simulink model "case3"  (R2024b)
settings: Solver=FixedStepAuto  StartTime=0  StopTime=1  FixedStep=1e-7  RelTol=1e-3
values from neighbouring files (symbols this model uses):
  SG_D_1_D = 0.01056    [IEEE9_case_parameters.m]    (also in case1_parameters.m; case2_parameters.m; case3_parameters.m; case4_parameters.m)
  SG_D_1_EnableSaturation = 0    [IEEE9_case_parameters.m]    (also in case1_parameters.m; case2_parameters.m; case3_parameters.m; case4_parameters.m)
  SG_D_1_f0 = 60    [IEEE9_case_parameters.m]    (also in case1_parameters.m; case2_parameters.m; case3_parameters.m; case4_parameters.m)
  SG_D_1_H = 7.5    [IEEE9_case_parameters.m]    (also in case1_parameters.m; case2_parameters.m; case3_parameters.m; case4_parameters.m)
  SG_D_1_K_A = 20    [IEEE9_case_parameters.m]    (also in case1_parameters.m; case2_parameters.m; case3_parameters.m; case4_parameters.m)
  SG_D_1_K_E = 1.000000e+1    (= 10)    [IEEE9_case_parameters.m]    (also in case1_parameters.m; case2_parameters.m; case3_parameters.m; case4_parameters.m)
  SG_D_1_K_F = 2.363    [IEEE9_case_parameters.m]    (also in case1_parameters.m; case2_parameters.m; case3_parameters.m; case4_parameters.m)
  SG_D_1_K_s = 0.5    [IEEE9_case_parameters.m]    (also in case1_parameters.m = 5; case2_parameters.m = 5; case3_parameters.m = 5; case4_parameters.m = 5)
  SG_D_1_R_a = 0.001088    [IEEE9_case_parameters.m]    (also in case1_parameters.m; case2_parameters.m; case3_parameters.m; case4_parameters.m)
  SG_D_1_S_A = 1    [IEEE9_case_parameters.m]    (also in case1_parameters.m; case2_parameters.m; case3_parameters.m; case4_parameters.m)
  SG_D_1_S_B = 0.103    [IEEE9_case_parameters.m]    (also in case1_parameters.m; case2_parameters.m; case3_parameters.m; case4_parameters.m)
  SG_D_1_S_N = 10.659857    [IEEE9_case_parameters.m]    (also in case1_parameters.m; case2_parameters.m; case3_parameters.m; case4_parameters.m)
  SG_D_1_SpeedPara = 200    [IEEE9_case_parameters.m]    (also in case1_parameters.m; case2_parameters.m; case3_parameters.m; case4_parameters.m)
  SG_D_1_T_0 = 0.720173    [IEEE9_case_parameters.m]    (also in case1_parameters.m = 0.755522; case2_parameters.m = 0.808931; case3_parameters.m = 0.869402; case4_parameters.m = 0.729316)
  SG_D_1_T_1 = 0.3    [IEEE9_case_parameters.m]    (also in case1_parameters.m; case2_parameters.m; case3_parameters.m; case4_parameters.m)
  SG_D_1_T_2 = 0.05    [IEEE9_case_parameters.m]    (also in case1_parameters.m; case2_parameters.m; case3_parameters.m; case4_parameters.m)
  SG_D_1_T_3 = 0.02    [IEEE9_case_parameters.m]    (also in case1_parameters.m; case2_parameters.m; case3_parameters.m; case4_parameters.m)
  SG_D_1_T_4 = 0.005    [IEEE9_case_parameters.m]    (also in case1_parameters.m; case2_parameters.m; case3_parameters.m; case4_parameters.m)
  SG_D_1_T_A = 0.02    [IEEE9_case_parameters.m]    (also in case1_parameters.m; case2_parameters.m; case3_parameters.m; case4_parameters.m)
  SG_D_1_T_dd = 8.000000e+0    (= 8)    [IEEE9_case_parameters.m]    (also in case1_parameters.m; case2_parameters.m; case3_parameters.m; case4_parameters.m)
  SG_D_1_T_ddd = 0.04    [IEEE9_case_parameters.m]    (also in case1_parameters.m; case2_parameters.m; case3_parameters.m; case4_parameters.m)
  SG_D_1_T_E = 0.314    [IEEE9_case_parameters.m]    (also in case1_parameters.m; case2_parameters.m; case3_parameters.m; case4_parameters.m)
  SG_D_1_T_F = 0.35    [IEEE9_case_parameters.m]    (also in case1_parameters.m; case2_parameters.m; case3_parameters.m; case4_parameters.m)
  SG_D_1_T_qd = 0.8    [IEEE9_case_parameters.m]    (also in case1_parameters.m; case2_parameters.m; case3_parameters.m; case4_parameters.m)
  SG_D_1_T_qdd = 0.02    [IEEE9_case_parameters.m]    (also in case1_parameters.m; case2_parameters.m; case3_parameters.m; case4_parameters.m)
  SG_D_1_T_speed = 0.1    [IEEE9_case_parameters.m]    (also in case1_parameters.m = 200; case2_parameters.m = 200; case3_parameters.m = 200; case4_parameters.m = 200)
  SG_D_1_T_w = 0.5    [IEEE9_case_parameters.m]    (also in case1_parameters.m; case2_parameters.m; case3_parameters.m; case4_parameters.m)
  SG_D_1_V_ref = 1.990276    [IEEE9_case_parameters.m]    (also in case1_parameters.m = 2.042296; case2_parameters.m = 2.051388; case3_parameters.m = 2.089584; case4_parameters.m = 2.01845)
  SG_D_1_w_ref = 376.991118    [IEEE9_case_parameters.m]    (also in case1_parameters.m; case2_parameters.m; case3_parameters.m; case4_parameters.m)
  SG_D_1_wb = 6.000000e+1    (= 60)    [IEEE9_case_parameters.m]    (also in case1_parameters.m; case2_parameters.m; case3_parameters.m; case4_parameters.m)
  SG_D_1_x_d = 1.9    [IEEE9_case_parameters.m]    (also in case1_parameters.m; case2_parameters.m; case3_parameters.m; case4_parameters.m)
  SG_D_1_x_dd = 0.302    [IEEE9_case_parameters.m]    (also in case1_parameters.m; case2_parameters.m; case3_parameters.m; case4_parameters.m)
  SG_D_1_x_ddd = 0.204    [IEEE9_case_parameters.m]    (also in case1_parameters.m; case2_parameters.m; case3_parameters.m; case4_parameters.m)
  SG_D_1_x_l = 0.05    [IEEE9_case_parameters.m]    (also in case1_parameters.m; case2_parameters.m; case3_parameters.m; case4_parameters.m)
  SG_D_1_x_q = 1.3    [IEEE9_case_parameters.m]    (also in case1_parameters.m; case2_parameters.m; case3_parameters.m; case4_parameters.m)
  SG_D_1_x_qd = 0.5    [IEEE9_case_parameters.m]    (also in case1_parameters.m; case2_parameters.m; case3_parameters.m; case4_parameters.m)
  SG_D_1_x_qdd = 0.3    [IEEE9_case_parameters.m]    (also in case1_parameters.m; case2_parameters.m; case3_parameters.m; case4_parameters.m)
  SG_D_2_D = 0.02    [IEEE9_case_parameters.m]    (also in case1_parameters.m; case2_parameters.m; case3_parameters.m; case4_parameters.m)
  SG_D_2_EnableSaturation = 0    [IEEE9_case_parameters.m]    (also in case1_parameters.m; case2_parameters.m; case3_parameters.m; case4_parameters.m)
  SG_D_2_f0 = 60    [IEEE9_case_parameters.m]    (also in case1_parameters.m; case2_parameters.m; case3_parameters.m; case4_parameters.m)
  SG_D_2_H = 8.000000e+0    (= 8)    [IEEE9_case_parameters.m]    (also in case1_parameters.m; case2_parameters.m; case3_parameters.m; case4_parameters.m)
  SG_D_2_K_A = 20    [IEEE9_case_parameters.m]    (also in case1_parameters.m; case2_parameters.m; case3_parameters.m; case4_parameters.m)
  SG_D_2_K_E = 1.000000e+1    (= 10)    [IEEE9_case_parameters.m]    (also in case1_parameters.m; case2_parameters.m; case3_parameters.m; case4_parameters.m)
  SG_D_2_K_F = 2.363    [IEEE9_case_parameters.m]    (also in case1_parameters.m; case2_parameters.m; case3_parameters.m; case4_parameters.m)
  SG_D_2_K_s = 0.5    [IEEE9_case_parameters.m]    (also in case1_parameters.m = 4; case2_parameters.m = 4; case3_parameters.m = 4; case4_parameters.m = 4)
  SG_D_2_R_a = 0.001088    [IEEE9_case_parameters.m]    (also in case1_parameters.m; case2_parameters.m; case3_parameters.m; case4_parameters.m)
  SG_D_2_S_A = 1    [IEEE9_case_parameters.m]    (also in case1_parameters.m; case2_parameters.m; case3_parameters.m; case4_parameters.m)
  SG_D_2_S_B = 0.103    [IEEE9_case_parameters.m]    (also in case1_parameters.m; case2_parameters.m; case3_parameters.m; case4_parameters.m)
  SG_D_2_S_N = 10.659857    [IEEE9_case_parameters.m]    (also in case1_parameters.m; case2_parameters.m; case3_parameters.m; case4_parameters.m)
  SG_D_2_SpeedPara = 200    [IEEE9_case_parameters.m]    (also in case1_parameters.m; case2_parameters.m; case3_parameters.m; case4_parameters.m)
  SG_D_2_T_0 = 1.632913    [IEEE9_case_parameters.m]    (also in case1_parameters.m = 1.632925; case2_parameters.m = 1.632915; case3_parameters.m = 1.632914; case4_parameters.m = 1.632927)
  SG_D_2_T_1 = 0.2    [IEEE9_case_parameters.m]    (also in case1_parameters.m; case2_parameters.m; case3_parameters.m; case4_parameters.m)
  SG_D_2_T_2 = 0.05    [IEEE9_case_parameters.m]    (also in case1_parameters.m; case2_parameters.m; case3_parameters.m; case4_parameters.m)
  SG_D_2_T_3 = 0.02    [IEEE9_case_parameters.m]    (also in case1_parameters.m; case2_parameters.m; case3_parameters.m; case4_parameters.m)
  SG_D_2_T_4 = 0.005    [IEEE9_case_parameters.m]    (also in case1_parameters.m; case2_parameters.m; case3_parameters.m; case4_parameters.m)
  SG_D_2_T_A = 0.02    [IEEE9_case_parameters.m]    (also in case1_parameters.m; case2_parameters.m; case3_parameters.m; case4_parameters.m)
  SG_D_2_T_dd = 7.9    [IEEE9_case_parameters.m]    (also in case1_parameters.m; case2_parameters.m; case3_parameters.m; case4_parameters.m)
  SG_D_2_T_ddd = 0.04    [IEEE9_case_parameters.m]    (also in case1_parameters.m; case2_parameters.m; case3_parameters.m; case4_parameters.m)
  SG_D_2_T_E = 0.314    [IEEE9_case_parameters.m]    (also in case1_parameters.m; case2_parameters.m; case3_parameters.m; case4_parameters.m)
  SG_D_2_T_F = 0.35    [IEEE9_case_parameters.m]    (also in case1_parameters.m; case2_parameters.m; case3_parameters.m; case4_parameters.m)
  SG_D_2_T_qd = 0.8    [IEEE9_case_parameters.m]    (also in case1_parameters.m; case2_parameters.m; case3_parameters.m; case4_parameters.m)
  SG_D_2_T_qdd = 0.015    [IEEE9_case_parameters.m]    (also in case1_parameters.m; case2_parameters.m; case3_parameters.m; case4_parameters.m)
  SG_D_2_T_speed = 0.1    [IEEE9_case_parameters.m]    (also in case1_parameters.m = 150; case2_parameters.m = 150; case3_parameters.m = 150; case4_parameters.m = 150)
  SG_D_2_T_w = 0.35    [IEEE9_case_parameters.m]    (also in case1_parameters.m; case2_parameters.m; case3_parameters.m; case4_parameters.m)
  SG_D_2_V_ref = 2.58547    [IEEE9_case_parameters.m]    (also in case1_parameters.m = 2.597896; case2_parameters.m = 2.587136; case3_parameters.m = 2.586042; case4_parameters.m = 2.599679)
  SG_D_2_w_ref = 376.991118    [IEEE9_case_parameters.m]    (also in case1_parameters.m; case2_parameters.m; case3_parameters.m; case4_parameters.m)
  SG_D_2_wb = 6.000000e+1    (= 60)    [IEEE9_case_parameters.m]    (also in case1_parameters.m; case2_parameters.m; case3_parameters.m; case4_parameters.m)
  SG_D_2_x_d = 1.8    [IEEE9_case_parameters.m]    (also in case1_parameters.m; case2_parameters.m; case3_parameters.m; case4_parameters.m)
  SG_D_2_x_dd = 0.302    [IEEE9_case_parameters.m]    (also in case1_parameters.m; case2_parameters.m; case3_parameters.m; case4_parameters.m)
  SG_D_2_x_ddd = 0.204    [IEEE9_case_parameters.m]    (also in case1_parameters.m; case2_parameters.m; case3_parameters.m; case4_parameters.m)
  SG_D_2_x_l = 0.05    [IEEE9_case_parameters.m]    (also in case1_parameters.m; case2_parameters.m; case3_parameters.m; case4_parameters.m)
  SG_D_2_x_q = 1.25    [IEEE9_case_parameters.m]    (also in case1_parameters.m; case2_parameters.m; case3_parameters.m; case4_parameters.m)
  SG_D_2_x_qd = 0.5    [IEEE9_case_parameters.m]    (also in case1_parameters.m; case2_parameters.m; case3_parameters.m; case4_parameters.m)
  SG_D_2_x_qdd = 0.3    [IEEE9_case_parameters.m]    (also in case1_parameters.m; case2_parameters.m; case3_parameters.m; case4_parameters.m)
  SG_D_3_D = 0.02    [IEEE9_case_parameters.m]    (also in case1_parameters.m; case2_parameters.m; case3_parameters.m; case4_parameters.m)
  SG_D_3_EnableSaturation = 0    [IEEE9_case_parameters.m]    (also in case1_parameters.m; case2_parameters.m; case3_parameters.m; case4_parameters.m)
  SG_D_3_f0 = 60    [IEEE9_case_parameters.m]    (also in case1_parameters.m; case2_parameters.m; case3_parameters.m; case4_parameters.m)
  SG_D_3_H = 7.7    [IEEE9_case_parameters.m]    (also in case1_parameters.m; case2_parameters.m; case3_parameters.m; case4_parameters.m)
  SG_D_3_K_A = 20    [IEEE9_case_parameters.m]    (also in case1_parameters.m; case2_parameters.m; case3_parameters.m; case4_parameters.m)
  SG_D_3_K_E = 1.000000e+1    (= 10)    [IEEE9_case_parameters.m]    (also in case1_parameters.m; case2_parameters.m; case3_parameters.m; case4_parameters.m)
  SG_D_3_K_F = 2.363    [IEEE9_case_parameters.m]    (also in case1_parameters.m; case2_parameters.m; case3_parameters.m; case4_parameters.m)
  SG_D_3_K_s = 0.2    [IEEE9_case_parameters.m]    (also in case1_parameters.m = 2; case2_parameters.m = 2; case3_parameters.m = 2; case4_parameters.m = 2)
  SG_D_3_R_a = 0.001088    [IEEE9_case_parameters.m]    (also in case1_parameters.m; case2_parameters.m; case3_parameters.m; case4_parameters.m)
  SG_D_3_S_A = 1    [IEEE9_case_parameters.m]    (also in case1_parameters.m; case2_parameters.m; case3_parameters.m; case4_parameters.m)
  SG_D_3_S_B = 0.103    [IEEE9_case_parameters.m]    (also in case1_parameters.m; case2_parameters.m; case3_parameters.m; case4_parameters.m)
  SG_D_3_S_N = 10.659857    [IEEE9_case_parameters.m]    (also in case1_parameters.m; case2_parameters.m; case3_parameters.m; case4_parameters.m)
  SG_D_3_SpeedPara = 200    [IEEE9_case_parameters.m]    (also in case1_parameters.m; case2_parameters.m; case3_parameters.m; case4_parameters.m)
  SG_D_3_T_0 = 0.850788    [IEEE9_case_parameters.m]    (also in case1_parameters.m = 0.850786; case2_parameters.m = 0.850787; case3_parameters.m; case4_parameters.m = 0.850786)
  SG_D_3_T_1 = 0.2    [IEEE9_case_parameters.m]    (also in case1_parameters.m; case2_parameters.m; case3_parameters.m; case4_parameters.m)
  SG_D_3_T_2 = 0.05    [IEEE9_case_parameters.m]    (also in case1_parameters.m; case2_parameters.m; case3_parameters.m; case4_parameters.m)
  SG_D_3_T_3 = 0.02    [IEEE9_case_parameters.m]    (also in case1_parameters.m; case2_parameters.m; case3_parameters.m; case4_parameters.m)
  SG_D_3_T_4 = 0.005    [IEEE9_case_parameters.m]    (also in case1_parameters.m; case2_parameters.m; case3_parameters.m; case4_parameters.m)
  SG_D_3_T_A = 0.02    [IEEE9_case_parameters.m]    (also in case1_parameters.m; case2_parameters.m; case3_parameters.m; case4_parameters.m)
  SG_D_3_T_dd = 8.1    [IEEE9_case_parameters.m]    (also in case1_parameters.m; case2_parameters.m; case3_parameters.m; case4_parameters.m)
  SG_D_3_T_ddd = 0.04    [IEEE9_case_parameters.m]    (also in case1_parameters.m; case2_parameters.m; case3_parameters.m; case4_parameters.m)
  SG_D_3_T_E = 0.314    [IEEE9_case_parameters.m]    (also in case1_parameters.m; case2_parameters.m; case3_parameters.m; case4_parameters.m)
  SG_D_3_T_F = 0.35    [IEEE9_case_parameters.m]    (also in case1_parameters.m; case2_parameters.m; case3_parameters.m; case4_parameters.m)
  SG_D_3_T_qd = 0.8    [IEEE9_case_parameters.m]    (also in case1_parameters.m; case2_parameters.m; case3_parameters.m; case4_parameters.m)
  SG_D_3_T_qdd = 0.015    [IEEE9_case_parameters.m]    (also in case1_parameters.m; case2_parameters.m; case3_parameters.m; case4_parameters.m)
  SG_D_3_T_speed = 0.1    [IEEE9_case_parameters.m]    (also in case1_parameters.m = 180; case2_parameters.m = 180; case3_parameters.m = 180; case4_parameters.m = 180)
  SG_D_3_T_w = 0.4    [IEEE9_case_parameters.m]    (also in case1_parameters.m; case2_parameters.m; case3_parameters.m; case4_parameters.m)
  SG_D_3_V_ref = 1.892727    [IEEE9_case_parameters.m]    (also in case1_parameters.m = 1.906439; case2_parameters.m = 1.895535; case3_parameters.m = 1.892105; case4_parameters.m = 1.906598)
  SG_D_3_w_ref = 376.991118    [IEEE9_case_parameters.m]    (also in case1_parameters.m; case2_parameters.m; case3_parameters.m; case4_parameters.m)
  SG_D_3_wb = 6.000000e+1    (= 60)    [IEEE9_case_parameters.m]    (also in case1_parameters.m; case2_parameters.m; case3_parameters.m; case4_parameters.m)
  SG_D_3_x_d = 1.85    [IEEE9_case_parameters.m]    (also in case1_parameters.m; case2_parameters.m; case3_parameters.m; case4_parameters.m)
  SG_D_3_x_dd = 0.302    [IEEE9_case_parameters.m]    (also in case1_parameters.m; case2_parameters.m; case3_parameters.m; case4_parameters.m)
  SG_D_3_x_ddd = 0.204    [IEEE9_case_parameters.m]    (also in case1_parameters.m; case2_parameters.m; case3_parameters.m; case4_parameters.m)
  SG_D_3_x_l = 0.05    [IEEE9_case_parameters.m]    (also in case1_parameters.m; case2_parameters.m; case3_parameters.m; case4_parameters.m)
  SG_D_3_x_q = 1.2    [IEEE9_case_parameters.m]    (also in case1_parameters.m; case2_parameters.m; case3_parameters.m; case4_parameters.m)
  SG_D_3_x_qd = 0.5    [IEEE9_case_parameters.m]    (also in case1_parameters.m; case2_parameters.m; case3_parameters.m; case4_parameters.m)
  SG_D_3_x_qdd = 0.3    [IEEE9_case_parameters.m]    (also in case1_parameters.m; case2_parameters.m; case3_parameters.m; case4_parameters.m)
(part 1 of 12)
settings Model: Creator=Greg  LastModifiedBy=Greg

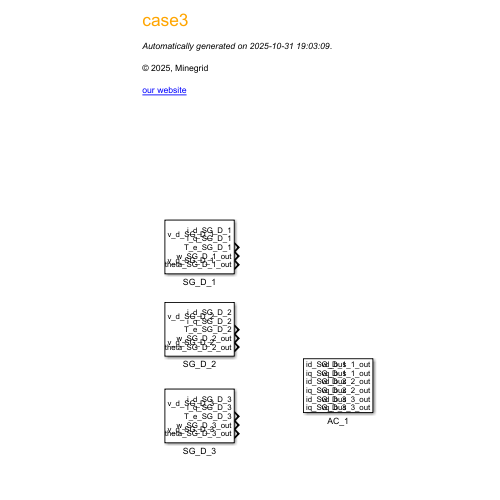
[thumbnail: Simulink's stored preview of the top-level diagram]
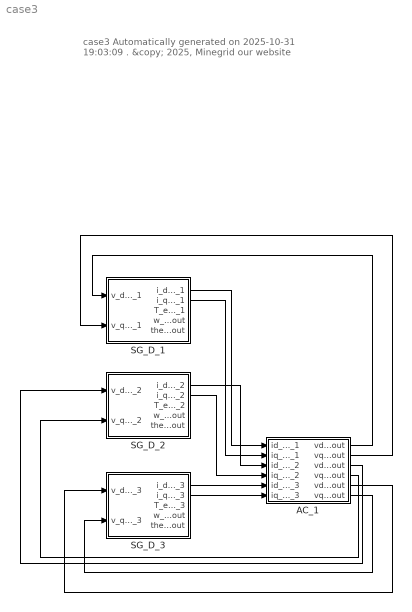
== system case3 ==
  note: case3
      | Automatically generated on 2025-10-31 19:03:09 .
      | &copy; 2025, Minegrid
      | our website
  AC_1 : Subsystem  mask(AC_1){}
      mask help: Parameters Interface of AC_1
  SG_D_1 : Subsystem  mask(SG_D_1){T_0=SG_D_1_T_0, w_ref=SG_D_1_w_ref, V_ref=SG_D_1_V_ref, x_d=SG_D_1_x_d, x_dd=SG_D_1_x_dd, x_ddd=SG_D_1_x_ddd, x_q=SG_D_1_x_q, x_qd=SG_D_1_x_qd, x_qdd=SG_D_1_x_qdd, x_l=SG_D_1_x_l, R_a=SG_D_1_R_a, T_dd=SG_D_1_T_dd, T_ddd=SG_D_1_T_ddd, T_qd=SG_D_1_T_qd, T_qdd=SG_D_1_T_qdd, H=SG_D_1_H, D=SG_D_1_D, SpeedPara=SG_D_1_SpeedPara, K_A=SG_D_1_K_A, EnableSaturation=SG_D_1_EnableSaturation, f0=SG_D_1_f0, T_speed=SG_D_1_T_speed, T_E=SG_D_1_T_E, T_A=SG_D_1_T_A, T_F=SG_D_1_T_F, K_E=SG_D_1_K_E, K_F=SG_D_1_K_F, K_s=SG_D_1_K_s, T_1=SG_D_1_T_1, T_2=SG_D_1_T_2, T_3=SG_D_1_T_3, T_4=SG_D_1_T_4, T_w=SG_D_1_T_w, wb=SG_D_1_wb, S_A=SG_D_1_S_A, S_B=SG_D_1_S_B, S_N=SG_D_1_S_N}
      mask help: Parameters Interface of SG_D_1
  SG_D_2 : Subsystem  mask(SG_D_2){T_0=SG_D_2_T_0, w_ref=SG_D_2_w_ref, V_ref=SG_D_2_V_ref, x_d=SG_D_2_x_d, x_dd=SG_D_2_x_dd, x_ddd=SG_D_2_x_ddd, x_q=SG_D_2_x_q, x_qd=SG_D_2_x_qd, x_qdd=SG_D_2_x_qdd, x_l=SG_D_2_x_l, R_a=SG_D_2_R_a, T_dd=SG_D_2_T_dd, T_ddd=SG_D_2_T_ddd, T_qd=SG_D_2_T_qd, T_qdd=SG_D_2_T_qdd, H=SG_D_2_H, D=SG_D_2_D, SpeedPara=SG_D_2_SpeedPara, K_A=SG_D_2_K_A, EnableSaturation=SG_D_2_EnableSaturation, f0=SG_D_2_f0, T_speed=SG_D_2_T_speed, T_E=SG_D_2_T_E, T_A=SG_D_2_T_A, T_F=SG_D_2_T_F, K_E=SG_D_2_K_E, K_F=SG_D_2_K_F, K_s=SG_D_2_K_s, T_1=SG_D_2_T_1, T_2=SG_D_2_T_2, T_3=SG_D_2_T_3, T_4=SG_D_2_T_4, T_w=SG_D_2_T_w, wb=SG_D_2_wb, S_A=SG_D_2_S_A, S_B=SG_D_2_S_B, S_N=SG_D_2_S_N}
      mask help: Parameters Interface of SG_D_2
  SG_D_3 : Subsystem  mask(SG_D_3){T_0=SG_D_3_T_0, w_ref=SG_D_3_w_ref, V_ref=SG_D_3_V_ref, x_d=SG_D_3_x_d, x_dd=SG_D_3_x_dd, x_ddd=SG_D_3_x_ddd, x_q=SG_D_3_x_q, x_qd=SG_D_3_x_qd, x_qdd=SG_D_3_x_qdd, x_l=SG_D_3_x_l, R_a=SG_D_3_R_a, T_dd=SG_D_3_T_dd, T_ddd=SG_D_3_T_ddd, T_qd=SG_D_3_T_qd, T_qdd=SG_D_3_T_qdd, H=SG_D_3_H, D=SG_D_3_D, SpeedPara=SG_D_3_SpeedPara, K_A=SG_D_3_K_A, EnableSaturation=SG_D_3_EnableSaturation, f0=SG_D_3_f0, T_speed=SG_D_3_T_speed, T_E=SG_D_3_T_E, T_A=SG_D_3_T_A, T_F=SG_D_3_T_F, K_E=SG_D_3_K_E, K_F=SG_D_3_K_F, K_s=SG_D_3_K_s, T_1=SG_D_3_T_1, T_2=SG_D_3_T_2, T_3=SG_D_3_T_3, T_4=SG_D_3_T_4, T_w=SG_D_3_T_w, wb=SG_D_3_wb, S_A=SG_D_3_S_A, S_B=SG_D_3_S_B, S_N=SG_D_3_S_N}
      mask help: Parameters Interface of SG_D_3
  wires:
  SG_D_2/2(i_q_SG_D_2) -> AC_1/4(iq_SG_D_2)
  SG_D_1/2(i_q_SG_D_1) -> AC_1/2(iq_SG_D_1)
  SG_D_1/1(i_d_SG_D_1) -> AC_1/1(id_SG_D_1)
  SG_D_2/1(i_d_SG_D_2) -> AC_1/3(id_SG_D_2)
  AC_1/1(vd_bus_1_out) -> SG_D_1/1(v_d_SG_D_1)
  SG_D_3/1(i_d_SG_D_3) -> AC_1/5(id_SG_D_3)
  AC_1/2(vq_bus_1_out) -> SG_D_1/2(v_q_SG_D_1)
  SG_D_3/2(i_q_SG_D_3) -> AC_1/6(iq_SG_D_3)
  AC_1/3(vd_bus_2_out) -> SG_D_2/1(v_d_SG_D_2)
  AC_1/4(vq_bus_2_out) -> SG_D_2/2(v_q_SG_D_2)
  AC_1/5(vd_bus_3_out) -> SG_D_3/1(v_d_SG_D_3)
  AC_1/6(vq_bus_3_out) -> SG_D_3/2(v_q_SG_D_3)

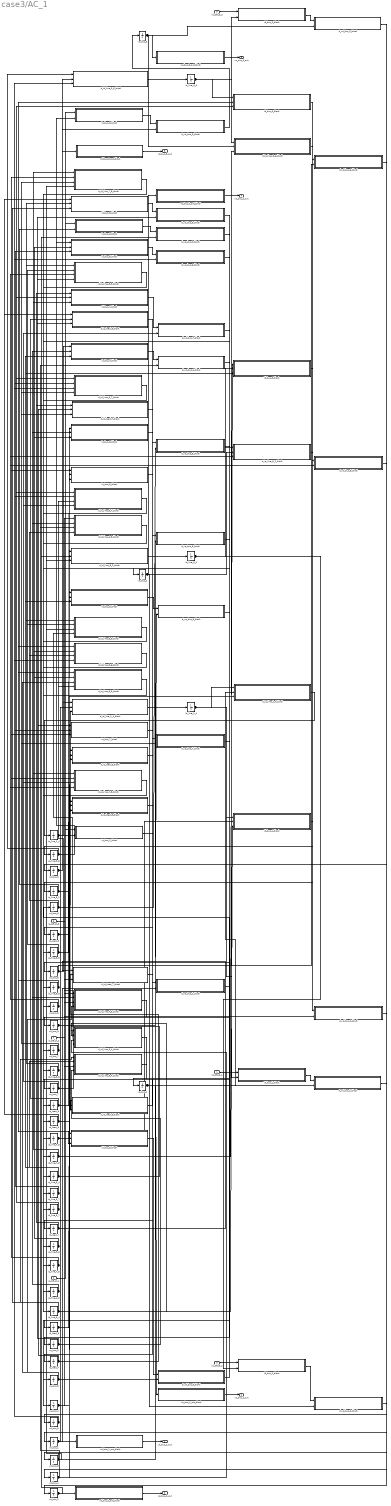
== system case3/AC_1 ==
  id_SG_D_1 : Inport
  iq_SG_D_1 : Inport  Port=2
  id_SG_D_2 : Inport  Port=3
  iq_SG_D_2 : Inport  Port=4
  id_SG_D_3 : Inport  Port=5
  iq_SG_D_3 : Inport  Port=6
  d_id_line_1_4_block : Subsystem
  d_id_line_3_6_block : Subsystem
  d_id_line_4_5_block : Subsystem
  d_id_line_5_6_block : Subsystem
  d_id_line_6_7_block : Subsystem
  d_id_line_7_8_block : Subsystem
  d_id_line_8_2_block : Subsystem
  d_id_line_8_9_block : Subsystem
  d_id_line_9_4_block : Subsystem
  d_id_load_5_block : Subsystem
  d_id_load_7_block : Subsystem
  d_id_load_9_block : Subsystem
  d_iq_line_1_4_block : Subsystem
  d_iq_line_3_6_block : Subsystem
  d_iq_line_4_5_block : Subsystem
  d_iq_line_5_6_block : Subsystem
  d_iq_line_6_7_block : Subsystem
  d_iq_line_7_8_block : Subsystem
  d_iq_line_8_2_block : Subsystem
  d_iq_line_8_9_block : Subsystem
  d_iq_line_9_4_block : Subsystem
  d_iq_load_5_block : Subsystem
  d_iq_load_7_block : Subsystem
  d_iq_load_9_block : Subsystem
  d_vd_bus_1_block : Subsystem
  d_vd_bus_2_block : Subsystem
  d_vd_bus_3_block : Subsystem
  d_vd_bus_4_block : Subsystem
  d_vd_bus_5_block : Subsystem
  d_vd_bus_6_block : Subsystem
  d_vd_bus_7_block : Subsystem
  d_vd_bus_8_block : Subsystem
  d_vd_bus_9_block : Subsystem
  d_vq_bus_1_block : Subsystem
  d_vq_bus_2_block : Subsystem
  d_vq_bus_3_block : Subsystem
  d_vq_bus_4_block : Subsystem
  d_vq_bus_5_block : Subsystem
  d_vq_bus_6_block : Subsystem
  d_vq_bus_7_block : Subsystem
  d_vq_bus_8_block : Subsystem
  d_vq_bus_9_block : Subsystem
  id_bus_1_block : Subsystem
  id_bus_2_block : Subsystem
  id_bus_3_block : Subsystem
  id_bus_4_block : Subsystem
  id_bus_5_block : Subsystem
  id_bus_6_block : Subsystem
  id_bus_7_block : Subsystem
  id_bus_8_block : Subsystem
  id_bus_9_block : Subsystem
  id_line_1_4 : Integrator  InitialCondition=0.8685
  id_line_3_6 : Integrator  InitialCondition=0.8456
  id_line_4_5 : Integrator  InitialCondition=0.3746
  id_line_5_6 : Integrator  InitialCondition=-0.5838
  id_line_6_7 : Integrator  InitialCondition=0.266
  id_line_7_8 : Integrator  InitialCondition=-0.7941
  id_line_8_2 : Integrator  InitialCondition=-1.633
  id_line_8_9 : Integrator  InitialCondition=0.8498
  id_line_9_4 : Integrator  InitialCondition=-0.4852
  id_load_5 : Integrator  InitialCondition=0.9359719094415446
  id_load_7 : Integrator  InitialCondition=1.058114773666789
  id_load_9 : Integrator  InitialCondition=1.3128275450508151
  iq_bus_1_block : Subsystem
  iq_bus_2_block : Subsystem
  iq_bus_3_block : Subsystem
  iq_bus_4_block : Subsystem
  iq_bus_5_block : Subsystem
  iq_bus_6_block : Subsystem
  iq_bus_7_block : Subsystem
  iq_bus_8_block : Subsystem
  iq_bus_9_block : Subsystem
  iq_line_1_4 : Integrator  InitialCondition=-0.239
  iq_line_3_6 : Integrator  InitialCondition=0.0944
  iq_line_4_5 : Integrator  InitialCondition=-0.0834
  iq_line_5_6 : Integrator  InitialCondition=0.0474
  iq_line_6_7 : Integrator  InitialCondition=-0.1426
  iq_line_7_8 : Integrator  InitialCondition=0.0351
  iq_line_8_2 : Integrator  InitialCondition=-0.1083
  iq_line_8_9 : Integrator  InitialCondition=-0.0829
  iq_line_9_4 : Integrator  InitialCondition=0.3203
  iq_load_5 : Integrator  InitialCondition=-0.3812628280514811
  iq_load_7 : Integrator  InitialCondition=-0.35410310514589904
  iq_load_9 : Integrator  InitialCondition=-0.6326059955985617
  vd_bus_1 : Integrator  InitialCondition=1.0
  vd_bus_1_out_block : Subsystem
  vd_bus_2 : Integrator  InitialCondition=0.9879091097107321
  vd_bus_2_out_block : Subsystem
  vd_bus_3 : Integrator  InitialCondition=0.9977645153986716
  vd_bus_3_out_block : Subsystem
  vd_bus_4 : Integrator  InitialCondition=0.9855935027057598
  vd_bus_5 : Integrator  InitialCondition=0.9707528693348056
  vd_bus_6 : Integrator  InitialCondition=1.003554613883012
  vd_bus_7 : Integrator  InitialCondition=0.9851223493487857
  vd_bus_8 : Integrator  InitialCondition=0.9949914819674712
  vd_bus_9 : Integrator  InitialCondition=0.9519187352878377
  vq_bus_1 : Integrator  InitialCondition=0.0
  vq_bus_1_out_block : Subsystem
  vq_bus_2 : Integrator  InitialCondition=0.1550341605922668
  vq_bus_2_out_block : Subsystem
  vq_bus_3 : Integrator  InitialCondition=0.06682792688131226
  vq_bus_3_out_block : Subsystem
  vq_bus_4 : Integrator  InitialCondition=-0.05234370307058784
  vq_bus_5 : Integrator  InitialCondition=-0.08688371657456954
  vq_bus_6 : Integrator  InitialCondition=0.014981980389526698
  vq_bus_7 : Integrator  InitialCondition=-0.011257511235524303
  vq_bus_8 : Integrator  InitialCondition=0.04824761170151553
  vq_bus_9 : Integrator  InitialCondition=-0.09206900230068515
  vd_bus_1_out : Outport
  vq_bus_1_out : Outport  Port=2
  vd_bus_2_out : Outport  Port=3
  vq_bus_2_out : Outport  Port=4
  vd_bus_3_out : Outport  Port=5
  vq_bus_3_out : Outport  Port=6
  wires:
  vq_bus_2_out_block/1(Blockout_vq_bus_2_out_740a9) -> vq_bus_2_out/1
  d_id_line_1_4_block/1(Blockout_d_id_line_1_4_f5e01) -> id_line_1_4/1
  iq_SG_D_3/1 -> iq_bus_3_block/1(Input_iq_SG_D_3_dee65)
  vq_bus_1/1 -> d_vd_bus_1_block/2(State_vq_bus_1_8af1f), d_iq_line_1_4_block/2(State_vq_bus_1_eaf9d), vq_bus_1_out_block/1(State_vq_bus_1_ac5cf)
  vd_bus_3_out_block/1(Blockout_vd_bus_3_out_036f2) -> vd_bus_3_out/1
  d_iq_line_8_2_block/1(Blockout_d_iq_line_8_2_aa3d3) -> iq_line_8_2/1
  d_vd_bus_4_block/1(Blockout_d_vd_bus_4_12eb5) -> vd_bus_4/1
  id_SG_D_3/1 -> id_bus_3_block/1(Input_id_SG_D_3_6c44f)
  id_SG_D_2/1 -> id_bus_2_block/1(Input_id_SG_D_2_bafef)
  vq_bus_3_out_block/1(Blockout_vq_bus_3_out_fa0c1) -> vq_bus_3_out/1
  iq_bus_8_block/1(Blockout_iq_bus_8_33408) -> d_vq_bus_8_block/1(Alge_iq_bus_8_0043b)
  iq_SG_D_2/1 -> iq_bus_2_block/1(Input_iq_SG_D_2_ed99c)
  id_SG_D_1/1 -> id_bus_1_block/1(Input_id_SG_D_1_696b1)
  id_bus_9_block/1(Blockout_id_bus_9_70dbc) -> d_vd_bus_9_block/1(Alge_id_bus_9_730d0)
  iq_SG_D_1/1 -> iq_bus_1_block/1(Input_iq_SG_D_1_691df)
  d_id_load_7_block/1(Blockout_d_id_load_7_3ef5e) -> id_load_7/1
  iq_bus_6_block/1(Blockout_iq_bus_6_95ebc) -> d_vq_bus_6_block/1(Alge_iq_bus_6_a58d3)
  id_bus_3_block/1(Blockout_id_bus_3_5b536) -> d_vd_bus_3_block/1(Alge_id_bus_3_439ad)
  id_bus_8_block/1(Blockout_id_bus_8_01350) -> d_vd_bus_8_block/1(Alge_id_bus_8_ebbc1)
  iq_bus_9_block/1(Blockout_iq_bus_9_4e4a2) -> d_vq_bus_9_block/1(Alge_iq_bus_9_e4ae9)
  id_load_9/1 -> d_id_load_9_block/1(State_id_load_9_00ea3), id_bus_9_block/1(State_id_load_9_08adc), d_iq_load_9_block/1(State_id_load_9_95b0f)
  id_bus_4_block/1(Blockout_id_bus_4_47d2f) -> d_vd_bus_4_block/1(Alge_id_bus_4_7068c)
  vd_bus_1_out_block/1(Blockout_vd_bus_1_out_2faa7) -> vd_bus_1_out/1
  vq_bus_1_out_block/1(Blockout_vq_bus_1_out_b4fc0) -> vq_bus_1_out/1
  id_bus_5_block/1(Blockout_id_bus_5_0f46c) -> d_vd_bus_5_block/1(Alge_id_bus_5_5e52c)
  iq_line_7_8/1 -> iq_bus_7_block/3(State_iq_line_7_8_95be5), iq_bus_8_block/1(State_iq_line_7_8_0aaeb), d_iq_line_7_8_block/2(State_iq_line_7_8_0ca45), d_id_line_7_8_block/2(State_iq_line_7_8_8ab2b)
  iq_bus_7_block/1(Blockout_iq_bus_7_bb486) -> d_vq_bus_7_block/1(Alge_iq_bus_7_9bcfd)
  vd_bus_6/1 -> d_id_line_5_6_block/4(State_vd_bus_6_02860), d_id_line_3_6_block/3(State_vd_bus_6_86153), d_id_line_6_7_block/3(State_vd_bus_6_9819c), d_vq_bus_6_block/2(State_vd_bus_6_2678b)
  iq_bus_2_block/1(Blockout_iq_bus_2_c2560) -> d_vq_bus_2_block/1(Alge_iq_bus_2_2abe7)
  d_vd_bus_3_block/1(Blockout_d_vd_bus_3_94704) -> vd_bus_3/1
  id_bus_7_block/1(Blockout_id_bus_7_20b6b) -> d_vd_bus_7_block/1(Alge_id_bus_7_2d419)
  id_bus_6_block/1(Blockout_id_bus_6_05d15) -> d_vd_bus_6_block/1(Alge_id_bus_6_24922)
  id_line_4_5/1 -> id_bus_4_block/2(State_id_line_4_5_71002), d_iq_line_4_5_block/1(State_id_line_4_5_24b18), d_id_line_4_5_block/1(State_id_line_4_5_125e0), id_bus_5_block/2(State_id_line_4_5_78e66)
  vd_bus_2_out_block/1(Blockout_vd_bus_2_out_79f6a) -> vd_bus_2_out/1
  id_line_9_4/1 -> d_id_line_9_4_block/1(State_id_line_9_4_02a1a), d_iq_line_9_4_block/1(State_id_line_9_4_af562), id_bus_4_block/3(State_id_line_9_4_dd8eb), id_bus_9_block/3(State_id_line_9_4_1728f)
  vq_bus_8/1 -> d_vd_bus_8_block/2(State_vq_bus_8_8405d), d_iq_line_7_8_block/4(State_vq_bus_8_3d863), d_iq_line_8_9_block/3(State_vq_bus_8_011bb), d_iq_line_8_2_block/3(State_vq_bus_8_3e61a)
  iq_bus_5_block/1(Blockout_iq_bus_5_d6d28) -> d_vq_bus_5_block/1(Alge_iq_bus_5_f83f1)
  id_line_6_7/1 -> id_bus_6_block/3(State_id_line_6_7_32134), d_id_line_6_7_block/1(State_id_line_6_7_3cec9), d_iq_line_6_7_block/1(State_id_line_6_7_cd5da), id_bus_7_block/2(State_id_line_6_7_64680)
  id_bus_2_block/1(Blockout_id_bus_2_bddd5) -> d_vd_bus_2_block/1(Alge_id_bus_2_0b6c0)
  iq_bus_4_block/1(Blockout_iq_bus_4_14ae7) -> d_vq_bus_4_block/1(Alge_iq_bus_4_f534f)
  iq_bus_3_block/1(Blockout_iq_bus_3_7f48b) -> d_vq_bus_3_block/1(Alge_iq_bus_3_adc3d)
  id_bus_1_block/1(Blockout_id_bus_1_4a65c) -> d_vd_bus_1_block/1(Alge_id_bus_1_f922c)
  iq_line_8_2/1 -> d_id_line_8_2_block/1(State_iq_line_8_2_c2450), iq_bus_2_block/2(State_iq_line_8_2_3621d), iq_bus_8_block/2(State_iq_line_8_2_60ac3)
  iq_bus_1_block/1(Blockout_iq_bus_1_cefb8) -> d_vq_bus_1_block/1(Alge_iq_bus_1_c886c)
  d_id_line_3_6_block/1(Blockout_d_id_line_3_6_3490b) -> id_line_3_6/1
  d_vq_bus_7_block/1(Blockout_d_vq_bus_7_00412) -> vq_bus_7/1
  id_line_5_6/1 -> id_bus_6_block/2(State_id_line_5_6_cc1e8), d_iq_line_5_6_block/1(State_id_line_5_6_f3a7a), id_bus_5_block/3(State_id_line_5_6_8fb3f), d_id_line_5_6_block/1(State_id_line_5_6_11d83)
  iq_line_6_7/1 -> d_iq_line_6_7_block/2(State_iq_line_6_7_f3824), iq_bus_6_block/3(State_iq_line_6_7_054b0), iq_bus_7_block/2(State_iq_line_6_7_03f81), d_id_line_6_7_block/2(State_iq_line_6_7_7db22)
  id_line_8_2/1 -> id_bus_2_block/2(State_id_line_8_2_6b5a6), id_bus_8_block/2(State_id_line_8_2_3e7ba), d_iq_line_8_2_block/1(State_id_line_8_2_73741)
  d_iq_line_9_4_block/1(Blockout_d_iq_line_9_4_72d66) -> iq_line_9_4/1
  d_id_line_9_4_block/1(Blockout_d_id_line_9_4_f8e36) -> id_line_9_4/1
  vq_bus_5/1 -> d_vd_bus_5_block/2(State_vq_bus_5_467f2), d_iq_load_5_block/3(State_vq_bus_5_03c1b), d_iq_line_5_6_block/3(State_vq_bus_5_6825f), d_iq_line_4_5_block/4(State_vq_bus_5_9ee14)
  d_id_line_8_2_block/1(Blockout_d_id_line_8_2_922a4) -> id_line_8_2/1
  iq_line_9_4/1 -> d_id_line_9_4_block/2(State_iq_line_9_4_819ce), iq_bus_4_block/3(State_iq_line_9_4_3e12c), iq_bus_9_block/3(State_iq_line_9_4_00fae), d_iq_line_9_4_block/2(State_iq_line_9_4_ffcdd)
  d_iq_load_9_block/1(Blockout_d_iq_load_9_b592d) -> iq_load_9/1
  vq_bus_7/1 -> d_vd_bus_7_block/2(State_vq_bus_7_8f28b), d_iq_line_6_7_block/4(State_vq_bus_7_d9bfc), d_iq_line_7_8_block/3(State_vq_bus_7_50286), d_iq_load_7_block/3(State_vq_bus_7_a3eff)
  vd_bus_7/1 -> d_vq_bus_7_block/2(State_vd_bus_7_2341e), d_id_load_7_block/3(State_vd_bus_7_6ab08), d_id_line_6_7_block/4(State_vd_bus_7_1ec6b), d_id_line_7_8_block/3(State_vd_bus_7_bda80)
  d_id_load_9_block/1(Blockout_d_id_load_9_781d1) -> id_load_9/1
  iq_line_8_9/1 -> d_id_line_8_9_block/2(State_iq_line_8_9_f80cf), iq_bus_9_block/2(State_iq_line_8_9_f042c), iq_bus_8_block/3(State_iq_line_8_9_6619f), d_iq_line_8_9_block/2(State_iq_line_8_9_96dc9)
  d_id_load_5_block/1(Blockout_d_id_load_5_20828) -> id_load_5/1
  d_vd_bus_7_block/1(Blockout_d_vd_bus_7_d7b36) -> vd_bus_7/1
  id_line_3_6/1 -> id_bus_3_block/2(State_id_line_3_6_571a6), id_bus_6_block/1(State_id_line_3_6_c6af3), d_iq_line_3_6_block/1(State_id_line_3_6_f6ca7)
  d_vq_bus_6_block/1(Blockout_d_vq_bus_6_50300) -> vq_bus_6/1
  iq_load_9/1 -> d_iq_load_9_block/2(State_iq_load_9_9ab5c), iq_bus_9_block/1(State_iq_load_9_56201), d_id_load_9_block/2(State_iq_load_9_29708)
  d_vd_bus_5_block/1(Blockout_d_vd_bus_5_bd9e5) -> vd_bus_5/1
  vd_bus_5/1 -> d_id_load_5_block/3(State_vd_bus_5_9c3f5), d_id_line_5_6_block/3(State_vd_bus_5_794d2), d_vq_bus_5_block/2(State_vd_bus_5_2a82f), d_id_line_4_5_block/4(State_vd_bus_5_31906)
  id_line_8_9/1 -> d_id_line_8_9_block/1(State_id_line_8_9_8f4c6), d_iq_line_8_9_block/1(State_id_line_8_9_642ba), id_bus_8_block/3(State_id_line_8_9_302ee), id_bus_9_block/2(State_id_line_8_9_ceed5)
  id_line_7_8/1 -> id_bus_8_block/1(State_id_line_7_8_e2cc9), d_id_line_7_8_block/1(State_id_line_7_8_104c2), d_iq_line_7_8_block/1(State_id_line_7_8_b4d16), id_bus_7_block/3(State_id_line_7_8_85cde)
  id_load_7/1 -> d_id_load_7_block/1(State_id_load_7_e043e), id_bus_7_block/1(State_id_load_7_37f76), d_iq_load_7_block/1(State_id_load_7_f43ef)
  iq_line_3_6/1 -> d_id_line_3_6_block/1(State_iq_line_3_6_ad0cd), iq_bus_3_block/2(State_iq_line_3_6_61dd2), iq_bus_6_block/1(State_iq_line_3_6_33d27)
  iq_line_5_6/1 -> d_id_line_5_6_block/2(State_iq_line_5_6_14e07), d_iq_line_5_6_block/2(State_iq_line_5_6_affd3), iq_bus_5_block/3(State_iq_line_5_6_c4019), iq_bus_6_block/2(State_iq_line_5_6_019c6)
  vq_bus_3/1 -> d_vd_bus_3_block/2(State_vq_bus_3_ac889), vq_bus_3_out_block/1(State_vq_bus_3_4ba96), d_iq_line_3_6_block/2(State_vq_bus_3_2a06c)
  iq_line_4_5/1 -> d_id_line_4_5_block/2(State_iq_line_4_5_cfaf0), d_iq_line_4_5_block/2(State_iq_line_4_5_05a1c), iq_bus_4_block/2(State_iq_line_4_5_adb37), iq_bus_5_block/2(State_iq_line_4_5_89bcd)
  vd_bus_9/1 -> d_vq_bus_9_block/2(State_vd_bus_9_0824c), d_id_line_8_9_block/4(State_vd_bus_9_a0458), d_id_line_9_4_block/4(State_vd_bus_9_a7a68), d_id_load_9_block/3(State_vd_bus_9_36e95)
  id_line_1_4/1 -> d_iq_line_1_4_block/1(State_id_line_1_4_1c233), id_bus_1_block/2(State_id_line_1_4_e72f3), id_bus_4_block/1(State_id_line_1_4_bd9f3)
  iq_line_1_4/1 -> d_id_line_1_4_block/1(State_iq_line_1_4_fc81e), iq_bus_1_block/2(State_iq_line_1_4_8b10a), iq_bus_4_block/1(State_iq_line_1_4_b88bb)
  iq_load_7/1 -> d_id_load_7_block/2(State_iq_load_7_eee0e), d_iq_load_7_block/2(State_iq_load_7_a1d5b), iq_bus_7_block/1(State_iq_load_7_960e8)
  vd_bus_2/1 -> d_id_line_8_2_block/2(State_vd_bus_2_982da), vd_bus_2_out_block/1(State_vd_bus_2_2714d), d_vq_bus_2_block/2(State_vd_bus_2_d00a9)
  vd_bus_4/1 -> d_vq_bus_4_block/2(State_vd_bus_4_6453c), d_id_line_1_4_block/3(State_vd_bus_4_baee6), d_id_line_9_4_block/3(State_vd_bus_4_32929), d_id_line_4_5_block/3(State_vd_bus_4_48529)
  iq_load_5/1 -> d_id_load_5_block/2(State_iq_load_5_e6e38), d_iq_load_5_block/2(State_iq_load_5_68fca), iq_bus_5_block/1(State_iq_load_5_2754d)
  id_load_5/1 -> d_id_load_5_block/1(State_id_load_5_21183), d_iq_load_5_block/1(State_id_load_5_e1948), id_bus_5_block/1(State_id_load_5_b6667)
  vq_bus_9/1 -> d_vd_bus_9_block/2(State_vq_bus_9_8a543), d_iq_load_9_block/3(State_vq_bus_9_4829d), d_iq_line_8_9_block/4(State_vq_bus_9_8381b), d_iq_line_9_4_block/4(State_vq_bus_9_46860)
  vd_bus_8/1 -> d_vq_bus_8_block/2(State_vd_bus_8_4778f), d_id_line_7_8_block/4(State_vd_bus_8_b8c1f), d_id_line_8_2_block/3(State_vd_bus_8_1a12f), d_id_line_8_9_block/3(State_vd_bus_8_789f7)
  vq_bus_6/1 -> d_vd_bus_6_block/2(State_vq_bus_6_63666), d_iq_line_3_6_block/3(State_vq_bus_6_a5f6f), d_iq_line_5_6_block/4(State_vq_bus_6_7d333), d_iq_line_6_7_block/3(State_vq_bus_6_01e40)
  vq_bus_4/1 -> d_iq_line_1_4_block/3(State_vq_bus_4_44892), d_vd_bus_4_block/2(State_vq_bus_4_69940), d_iq_line_4_5_block/3(State_vq_bus_4_3c986), d_iq_line_9_4_block/3(State_vq_bus_4_28404)
  vd_bus_1/1 -> d_vq_bus_1_block/2(State_vd_bus_1_0864e), d_id_line_1_4_block/2(State_vd_bus_1_32af8), vd_bus_1_out_block/1(State_vd_bus_1_379f4)
  vd_bus_3/1 -> d_vq_bus_3_block/2(State_vd_bus_3_4e169), d_id_line_3_6_block/2(State_vd_bus_3_f9f03), vd_bus_3_out_block/1(State_vd_bus_3_9218c)
  vq_bus_2/1 -> d_vd_bus_2_block/2(State_vq_bus_2_58237), d_iq_line_8_2_block/2(State_vq_bus_2_813db), vq_bus_2_out_block/1(State_vq_bus_2_9d425)
  d_vd_bus_1_block/1(Blockout_d_vd_bus_1_fbb6b) -> vd_bus_1/1
  d_iq_line_8_9_block/1(Blockout_d_iq_line_8_9_02383) -> iq_line_8_9/1
  d_iq_line_1_4_block/1(Blockout_d_iq_line_1_4_64f6a) -> iq_line_1_4/1
  d_iq_load_5_block/1(Blockout_d_iq_load_5_e65a1) -> iq_load_5/1
  d_id_line_5_6_block/1(Blockout_d_id_line_5_6_8629c) -> id_line_5_6/1
  d_id_line_4_5_block/1(Blockout_d_id_line_4_5_12103) -> id_line_4_5/1
  d_id_line_6_7_block/1(Blockout_d_id_line_6_7_d9830) -> id_line_6_7/1
  d_vq_bus_2_block/1(Blockout_d_vq_bus_2_6ba06) -> vq_bus_2/1
  d_id_line_7_8_block/1(Blockout_d_id_line_7_8_1308e) -> id_line_7_8/1
  d_id_line_8_9_block/1(Blockout_d_id_line_8_9_9c30d) -> id_line_8_9/1
  d_vd_bus_8_block/1(Blockout_d_vd_bus_8_98eda) -> vd_bus_8/1
  d_iq_line_3_6_block/1(Blockout_d_iq_line_3_6_89a9d) -> iq_line_3_6/1
  d_iq_line_4_5_block/1(Blockout_d_iq_line_4_5_2a670) -> iq_line_4_5/1
  d_iq_load_7_block/1(Blockout_d_iq_load_7_43a8a) -> iq_load_7/1
  d_iq_line_5_6_block/1(Blockout_d_iq_line_5_6_beac2) -> iq_line_5_6/1
  d_vd_bus_9_block/1(Blockout_d_vd_bus_9_9d4f1) -> vd_bus_9/1
  d_iq_line_6_7_block/1(Blockout_d_iq_line_6_7_3df17) -> iq_line_6_7/1
  d_iq_line_7_8_block/1(Blockout_d_iq_line_7_8_5ff90) -> iq_line_7_8/1
  d_vq_bus_3_block/1(Blockout_d_vq_bus_3_16c3e) -> vq_bus_3/1
  d_vd_bus_2_block/1(Blockout_d_vd_bus_2_67dfb) -> vd_bus_2/1
  d_vq_bus_9_block/1(Blockout_d_vq_bus_9_e5b12) -> vq_bus_9/1
  d_vq_bus_1_block/1(Blockout_d_vq_bus_1_6dae5) -> vq_bus_1/1
  d_vd_bus_6_block/1(Blockout_d_vd_bus_6_74d5d) -> vd_bus_6/1
  d_vq_bus_4_block/1(Blockout_d_vq_bus_4_cec24) -> vq_bus_4/1
  d_vq_bus_5_block/1(Blockout_d_vq_bus_5_ebd21) -> vq_bus_5/1
  d_vq_bus_8_block/1(Blockout_d_vq_bus_8_7125c) -> vq_bus_8/1

== system case3/SG_D_1 ==
  v_d_SG_D_1 : Inport
  v_q_SG_D_1 : Inport  Port=2
  E_fd_SG_D_1 : Integrator  InitialCondition=2.1791689937604724
  Px_1_SG_D_1 : Integrator  InitialCondition=0.0
  Px_2_SG_D_1 : Integrator  InitialCondition=0.0
  Px_3_SG_D_1 : Integrator  InitialCondition=1.446762563402067e-31
  R_f_SG_D_1 : Integrator  InitialCondition=14.712503806445705
  T_e_SG_D_1_block : Subsystem
  T_m_SG_D_1 : Integrator  InitialCondition=0.8694016480988188
  V_f_SG_D_1 : Integrator  InitialCondition=21.791689937604723
  d_E_fd_SG_D_1_block : Subsystem
  d_Px_1_SG_D_1_block : Subsystem
  d_Px_2_SG_D_1_block : Subsystem
  d_Px_3_SG_D_1_block : Subsystem
  d_R_f_SG_D_1_block : Subsystem
  d_T_m_SG_D_1_block : Subsystem
  d_V_f_SG_D_1_block : Subsystem
  d_psi_1d_SG_D_1_block : Subsystem
  d_psi_d_SG_D_1_block : Subsystem
  d_psi_fd_SG_D_1_block : Subsystem
  d_psi_gq_SG_D_1_block : Subsystem
  d_psi_kq_SG_D_1_block : Subsystem
  d_psi_q_SG_D_1_block : Subsystem
  d_theta_SG_D_1_block : Subsystem
  d_w_SG_D_1_block : Subsystem
  i_d_SG_D_1_block : Subsystem
  i_q_SG_D_1_block : Subsystem
  psi_1d_SG_D_1 : Integrator  InitialCondition=0.7959021034955275
  psi_d_SG_D_1 : Integrator  InitialCondition=0.7585165118667451
  psi_fd_SG_D_1 : Integrator  InitialCondition=0.9843254853045903
  psi_gq_SG_D_1 : Integrator  InitialCondition=0.4019095526107287
  psi_kq_SG_D_1 : Integrator  InitialCondition=-0.6279836759542635
  psi_q_SG_D_1 : Integrator  InitialCondition=-0.6531030229924341
  theta_SG_D_1 : Integrator  InitialCondition=0.7106011105047251
  theta_SG_D_1_out_block : Subsystem
  w_SG_D_1 : Integrator  InitialCondition=376.99111843077515
  w_SG_D_1_out_block : Subsystem
  i_d_SG_D_1 : Outport
  i_q_SG_D_1 : Outport  Port=2
  T_e_SG_D_1 : Outport  Port=3
  w_SG_D_1_out : Outport  Port=4
  theta_SG_D_1_out : Outport  Port=5
  wires:
  V_f_SG_D_1/1 -> d_V_f_SG_D_1_block/14(State_V_f_SG_D_1_546a3), d_E_fd_SG_D_1_block/2(State_V_f_SG_D_1_a5ff7)
  psi_kq_SG_D_1/1 -> d_psi_q_SG_D_1_block/2(State_psi_kq_SG_D_1_5e11c), d_psi_gq_SG_D_1_block/3(State_psi_kq_SG_D_1_e61df), d_psi_gq_SG_D_1_block/5(State_psi_kq_SG_D_1_ce16b), d_psi_kq_SG_D_1_block/4(State_psi_kq_SG_D_1_06d41), d_psi_kq_SG_D_1_block/2(State_psi_kq_SG_D_1_e445d), d_w_SG_D_1_block/5(State_psi_kq_SG_D_1_63f5c), i_d_SG_D_1_block/2(State_psi_kq_SG_D_1_04692), i_q_SG_D_1_block/2(State_psi_kq_SG_D_1_9d437), d_V_f_SG_D_1_block/10(State_psi_kq_SG_D_1_bfe07), d_psi_gq_SG_D_1_block/8(State_psi_kq_SG_D_1_335cf), T_e_SG_D_1_block/3(State_psi_kq_SG_D_1_043c6)
  w_SG_D_1_out_block/1(Blockout_w_SG_D_1_out_d9996) -> w_SG_D_1_out/1
  d_theta_SG_D_1_block/1(Blockout_d_theta_SG_D_1_4a614) -> theta_SG_D_1/1
  d_Px_1_SG_D_1_block/1(Blockout_d_Px_1_SG_D_1_2cd45) -> Px_1_SG_D_1/1
  w_SG_D_1/1 -> d_psi_q_SG_D_1_block/9(State_w_SG_D_1_cf84f), d_V_f_SG_D_1_block/8(State_w_SG_D_1_345f1), d_V_f_SG_D_1_block/13(State_w_SG_D_1_c9c32), d_theta_SG_D_1_block/1(State_w_SG_D_1_fb02a), d_Px_3_SG_D_1_block/6(State_w_SG_D_1_8f01a), d_Px_2_SG_D_1_block/4(State_w_SG_D_1_5fb1d), d_w_SG_D_1_block/1(State_w_SG_D_1_a6451), d_T_m_SG_D_1_block/1(State_w_SG_D_1_82698), w_SG_D_1_out_block/1(State_w_SG_D_1_fc530), d_psi_d_SG_D_1_block/9(State_w_SG_D_1_754af), d_Px_1_SG_D_1_block/2(State_w_SG_D_1_918fc)
  d_Px_3_SG_D_1_block/1(Blockout_d_Px_3_SG_D_1_c155d) -> Px_3_SG_D_1/1
  d_Px_2_SG_D_1_block/1(Blockout_d_Px_2_SG_D_1_b732b) -> Px_2_SG_D_1/1
  d_T_m_SG_D_1_block/1(Blockout_d_T_m_SG_D_1_21740) -> T_m_SG_D_1/1
  psi_gq_SG_D_1/1 -> d_psi_gq_SG_D_1_block/1(State_psi_gq_SG_D_1_62535), d_psi_gq_SG_D_1_block/2(State_psi_gq_SG_D_1_054f8), d_psi_q_SG_D_1_block/1(State_psi_gq_SG_D_1_d9645), d_psi_kq_SG_D_1_block/3(State_psi_gq_SG_D_1_b227a), d_w_SG_D_1_block/4(State_psi_gq_SG_D_1_95977), d_V_f_SG_D_1_block/9(State_psi_gq_SG_D_1_8fed2), i_d_SG_D_1_block/1(State_psi_gq_SG_D_1_06924), d_psi_kq_SG_D_1_block/1(State_psi_gq_SG_D_1_92ffe), i_q_SG_D_1_block/1(State_psi_gq_SG_D_1_d01d3), d_psi_gq_SG_D_1_block/7(State_psi_gq_SG_D_1_49cf1), d_psi_gq_SG_D_1_block/4(State_psi_gq_SG_D_1_2e6d2), T_e_SG_D_1_block/2(State_psi_gq_SG_D_1_4e0b7)
  psi_fd_SG_D_1/1 -> d_psi_fd_SG_D_1_block/7(State_psi_fd_SG_D_1_f98c2), d_psi_fd_SG_D_1_block/10(State_psi_fd_SG_D_1_13afa), d_psi_fd_SG_D_1_block/2(State_psi_fd_SG_D_1_d4fb7), d_psi_d_SG_D_1_block/3(State_psi_fd_SG_D_1_dc6ee), d_psi_fd_SG_D_1_block/4(State_psi_fd_SG_D_1_4440b), d_psi_1d_SG_D_1_block/5(State_psi_fd_SG_D_1_95a16), d_w_SG_D_1_block/10(State_psi_fd_SG_D_1_6708f), d_psi_1d_SG_D_1_block/2(State_psi_fd_SG_D_1_fedb2), d_V_f_SG_D_1_block/6(State_psi_fd_SG_D_1_ab597), i_d_SG_D_1_block/7(State_psi_fd_SG_D_1_d596f), T_e_SG_D_1_block/8(State_psi_fd_SG_D_1_be33b), i_q_SG_D_1_block/7(State_psi_fd_SG_D_1_33a9d)
  Px_1_SG_D_1/1 -> d_Px_1_SG_D_1_block/1(State_Px_1_SG_D_1_be173), d_Px_3_SG_D_1_block/4(State_Px_1_SG_D_1_0dee8), d_Px_3_SG_D_1_block/5(State_Px_1_SG_D_1_09b4d), d_Px_2_SG_D_1_block/3(State_Px_1_SG_D_1_e9c5b), d_Px_2_SG_D_1_block/2(State_Px_1_SG_D_1_0d618)
  v_d_SG_D_1/1 -> d_psi_q_SG_D_1_block/4(Input_v_d_SG_D_1_19fdc), d_psi_d_SG_D_1_block/4(Input_v_d_SG_D_1_d8586)
  v_q_SG_D_1/1 -> d_psi_d_SG_D_1_block/6(Input_v_q_SG_D_1_8ffea), d_psi_q_SG_D_1_block/6(Input_v_q_SG_D_1_e60b4)
  psi_q_SG_D_1/1 -> d_psi_d_SG_D_1_block/8(State_psi_q_SG_D_1_46dab), d_psi_q_SG_D_1_block/3(State_psi_q_SG_D_1_8b0a5), d_psi_gq_SG_D_1_block/9(State_psi_q_SG_D_1_b7060), d_psi_kq_SG_D_1_block/5(State_psi_q_SG_D_1_463f3), d_w_SG_D_1_block/7(State_psi_q_SG_D_1_c4891), i_d_SG_D_1_block/3(State_psi_q_SG_D_1_1a988), d_psi_gq_SG_D_1_block/6(State_psi_q_SG_D_1_6f016), d_w_SG_D_1_block/6(State_psi_q_SG_D_1_cb802), i_q_SG_D_1_block/3(State_psi_q_SG_D_1_8c0e7), d_V_f_SG_D_1_block/7(State_psi_q_SG_D_1_9d0d1), T_e_SG_D_1_block/4(State_psi_q_SG_D_1_aebda), T_e_SG_D_1_block/5(State_psi_q_SG_D_1_dfa5e), d_V_f_SG_D_1_block/11(State_psi_q_SG_D_1_19a3e)
  theta_SG_D_1/1 -> d_psi_d_SG_D_1_block/5(State_theta_SG_D_1_f81ae), d_psi_q_SG_D_1_block/5(State_theta_SG_D_1_3237f), d_psi_q_SG_D_1_block/7(State_theta_SG_D_1_9067a), i_d_SG_D_1_block/8(State_theta_SG_D_1_7475d), i_d_SG_D_1_block/4(State_theta_SG_D_1_ace1c), i_q_SG_D_1_block/4(State_theta_SG_D_1_2faf8), i_q_SG_D_1_block/8(State_theta_SG_D_1_efa60), theta_SG_D_1_out_block/1(State_theta_SG_D_1_c9680), d_psi_d_SG_D_1_block/7(State_theta_SG_D_1_ab80e)
  psi_d_SG_D_1/1 -> d_psi_q_SG_D_1_block/8(State_psi_d_SG_D_1_31d3d), d_psi_d_SG_D_1_block/2(State_psi_d_SG_D_1_ff70f), d_psi_fd_SG_D_1_block/6(State_psi_d_SG_D_1_2a109), d_psi_1d_SG_D_1_block/4(State_psi_d_SG_D_1_96939), d_w_SG_D_1_block/3(State_psi_d_SG_D_1_d3254), d_V_f_SG_D_1_block/12(State_psi_d_SG_D_1_44844), i_d_SG_D_1_block/6(State_psi_d_SG_D_1_ee150), d_V_f_SG_D_1_block/5(State_psi_d_SG_D_1_438e5), i_q_SG_D_1_block/6(State_psi_d_SG_D_1_f3b11), T_e_SG_D_1_block/1(State_psi_d_SG_D_1_3a885), d_psi_fd_SG_D_1_block/9(State_psi_d_SG_D_1_32ce4), d_w_SG_D_1_block/9(State_psi_d_SG_D_1_bbfc2), T_e_SG_D_1_block/7(State_psi_d_SG_D_1_bdeee)
  Px_2_SG_D_1/1 -> d_Px_2_SG_D_1_block/1(State_Px_2_SG_D_1_f7c33), d_Px_3_SG_D_1_block/2(State_Px_2_SG_D_1_d9c58), d_Px_3_SG_D_1_block/3(State_Px_2_SG_D_1_c3f1d)
  T_m_SG_D_1/1 -> d_T_m_SG_D_1_block/2(State_T_m_SG_D_1_b9754), d_w_SG_D_1_block/2(State_T_m_SG_D_1_caef1)
  d_E_fd_SG_D_1_block/1(Blockout_d_E_fd_SG_D_1_6015a) -> E_fd_SG_D_1/1
  psi_1d_SG_D_1/1 -> d_psi_fd_SG_D_1_block/3(State_psi_1d_SG_D_1_7112e), d_psi_fd_SG_D_1_block/5(State_psi_1d_SG_D_1_457d2), d_psi_fd_SG_D_1_block/8(State_psi_1d_SG_D_1_118f1), d_psi_d_SG_D_1_block/1(State_psi_1d_SG_D_1_32408), d_psi_1d_SG_D_1_block/1(State_psi_1d_SG_D_1_e272b), d_psi_1d_SG_D_1_block/3(State_psi_1d_SG_D_1_7d194), d_V_f_SG_D_1_block/4(State_psi_1d_SG_D_1_33379), i_d_SG_D_1_block/5(State_psi_1d_SG_D_1_017fc), i_q_SG_D_1_block/5(State_psi_1d_SG_D_1_0c5a6), T_e_SG_D_1_block/6(State_psi_1d_SG_D_1_26ac5), d_w_SG_D_1_block/8(State_psi_1d_SG_D_1_916d9)
  d_psi_1d_SG_D_1_block/1(Blockout_d_psi_1d_SG_D_1_9d8e2) -> psi_1d_SG_D_1/1
  i_q_SG_D_1_block/1(Blockout_i_q_SG_D_1_dd5f1) -> i_q_SG_D_1/1
  d_psi_d_SG_D_1_block/1(Blockout_d_psi_d_SG_D_1_c7dc2) -> psi_d_SG_D_1/1
  d_psi_kq_SG_D_1_block/1(Blockout_d_psi_kq_SG_D_1_a4a4a) -> psi_kq_SG_D_1/1
  d_V_f_SG_D_1_block/1(Blockout_d_V_f_SG_D_1_ca827) -> V_f_SG_D_1/1
  d_R_f_SG_D_1_block/1(Blockout_d_R_f_SG_D_1_eadac) -> R_f_SG_D_1/1
  d_psi_q_SG_D_1_block/1(Blockout_d_psi_q_SG_D_1_513bd) -> psi_q_SG_D_1/1
  T_e_SG_D_1_block/1(Blockout_T_e_SG_D_1_96ef2) -> T_e_SG_D_1/1
  i_d_SG_D_1_block/1(Blockout_i_d_SG_D_1_03b31) -> i_d_SG_D_1/1
  d_psi_gq_SG_D_1_block/1(Blockout_d_psi_gq_SG_D_1_d0b28) -> psi_gq_SG_D_1/1
  d_w_SG_D_1_block/1(Blockout_d_w_SG_D_1_c2c2b) -> w_SG_D_1/1
  theta_SG_D_1_out_block/1(Blockout_theta_SG_D_1_out_2820c) -> theta_SG_D_1_out/1
  R_f_SG_D_1/1 -> d_R_f_SG_D_1_block/2(State_R_f_SG_D_1_95d12), d_V_f_SG_D_1_block/2(State_R_f_SG_D_1_61cc8)
  Px_3_SG_D_1/1 -> d_V_f_SG_D_1_block/3(State_Px_3_SG_D_1_83c94), d_Px_3_SG_D_1_block/1(State_Px_3_SG_D_1_48de8)
  E_fd_SG_D_1/1 -> d_V_f_SG_D_1_block/1(State_E_fd_SG_D_1_4eb3f), d_E_fd_SG_D_1_block/1(State_E_fd_SG_D_1_54b5a), d_R_f_SG_D_1_block/1(State_E_fd_SG_D_1_a064f), d_psi_fd_SG_D_1_block/1(State_E_fd_SG_D_1_8527f)
  d_psi_fd_SG_D_1_block/1(Blockout_d_psi_fd_SG_D_1_186e8) -> psi_fd_SG_D_1/1
